simulink model "MPC"  (R2020b)
settings: Solver=ode45  StartTime=0.0  StopTime=1000  RelTol=1e-3  EnableMultiTasking=on
values from neighbouring files (symbols this model uses):
  adingain = [adingain 1 1 1 1 1]    [hwinit.m]
  adinoffs = [adinoffs 0 0 0 0 0]    [hwinit.m]
  daoutgain = 1*[-6]    [hwinit.m]
  daoutoffs = -[-0.0025]    [hwinit.m]
  Theta1_0 = pi    (= 3.14159265359)    [simulation.m]
  Theta2_0 = -pi/2    (= -1.57079632679)    [simulation.m]
  Thetad1_0 = 0    [simulation.m]
  Thetad2_0 = 0    [simulation.m]
undefined symbols (not defined in the file or in its folder): Discrete, h, R, Time
libraries: simulink x4, mpclib x2, ctrlSharedLib x1
settings Model: Creator=rbabuska  LastModifiedBy=fballast
settings DataIOCC: LimitDataPoints=on  SaveFormat=Array  ReturnWorkspaceOutputs=off  SignalLoggingName=sigsOut
settings OptimizationCC: BooleanDataType=off  ExpressionDepthLimit=2147483647  InitFltsAndDblsToZero=on  LifeSpan=inf
settings DebuggingCC: SaveWithParameterizedLinksMsg=none  SignalResolutionControl=TryResolveAllWithWarning  MultiTaskDSMMsg=warning  MultiTaskCondExecSysMsg=none  AllowSymbolicDim=off  StateNameClashWarn=warning  SFUnexpectedBacktrackingDiag=warning  SFNoUnconditionalDefaultTransitionDiag=warning  SFExecutionAtInitializationDiag=none  ArithmeticOperatorsInVariantConditions=warning
settings HardwareCC: ProdBitPerPointer=32  ProdBitPerSizeT=32  ProdBitPerPtrDiffT=32  ProdLargestAtomicFloat=None  ProdIntDivRoundTo=Undefined  ProdEndianess=Unspecified  ProdWordSize=32  ProdHWDeviceType=32-bit Generic  TargetUnknown=on
settings ModelReferenceCC: PropagateSignalLabelsOutOfModel=off
settings SFSimCC: SimUseLocalCustomCode=off  CustomCodeUndefinedFunction=UseInterfaceOnly
settings RTWCC: RTWUseLocalCustomCode=off
settings CodeAppCC: StateflowObjectComments=on
settings GRTTargetCC: TargetFcnLib=ansi_tfl_tmw.mat  TargetLangStandard=C89/C90 (ANSI)  CombineOutputUpdateFcns=off  GRTInterface=on
settings ConfigComp: CovMetricSettings=dw  CovSaveCumulativeToWorkspaceVar=on  CovSaveSingleToWorkspaceVar=on  CovExternalEMLEnable=off

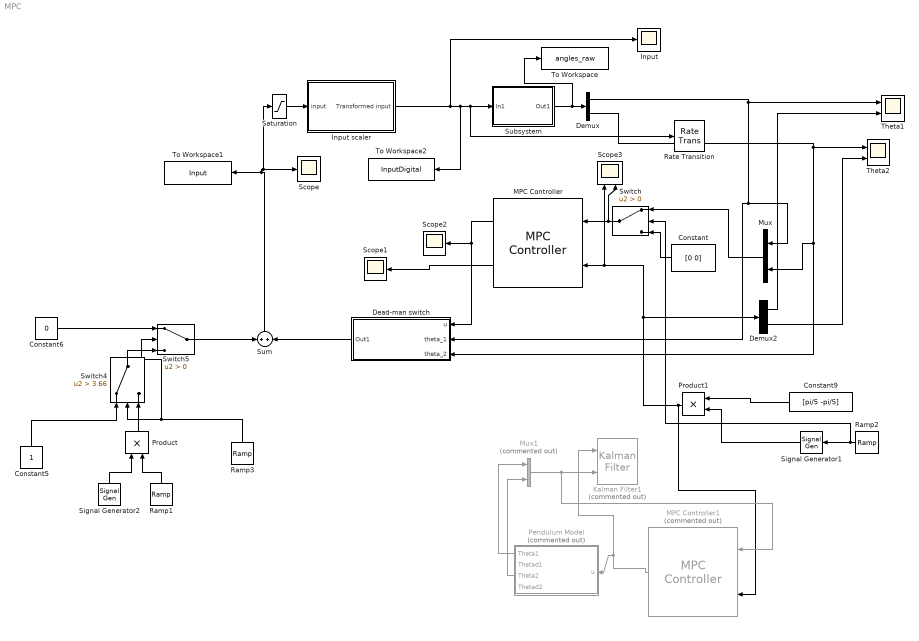
== system MPC ==
  Constant : Constant  Value=[0 0]
  Constant5 : Constant
  Constant6 : Constant  Value=0
  Constant9 : Constant  Value=[pi/5 -pi/5]
  Dead-man switch : Subsystem
  Demux : Demux  Outputs=2
  Demux2 : Demux  Outputs=2
  Input : Scope
  Input scaler : Subsystem
  Kalman Filter1 : ctrlSharedLib/Kalman Filter  Commented=on  TimeDomain=Discrete-Time  UseCurrentEstimator=on  ModelSource=LTI State-Space Variable  ModelSourceVariable=sysd  A=0.95  B=1  C=1  D=0  NumberOfStates=1  NumberOfInputs=1  NumberOfOutputs=1  InitialEstimateSource=Dialog  X0=0  P0=10  UseK=off  UseGH=off  NumberOfProcessNoiseInputs=1  G=eye(4)  TimeInvariantG=on  H=0  TimeInvariantH=on  Q=Q  TimeInvariantQ=on  R=R  TimeInvariantR=on  N=0  TimeInvariantN=on  AddInputPort=on  AddEnablePort=off  OutputEstimatedY=off  OutputP=off  Ts=-1
  MPC Controller : mpclib/MPC Controller  SCDEnableBlockLinearizationSpecification=on  mpcobj=mpc1  is_multiple=0  enable_value=0  return_u0=off  updateMPCinCallerWorkspace=on  md_inport=off  mv_inport=off  uref_inport=off  return_cost=off  return_mvseq=off  return_qpstatus=off  return_xseq=off  return_state=on  return_ovseq=off  state_inport=off  umin_inport=off  umax_inport=off  ymin_inport=off  ymax_inport=off  cc_inport=off  ywt_inport=off  uwt_inport=off  duwt_inport=off  rhoeps_inport=off  pm_inport=off  MaximumP=10  HorizonChoice=FixedHorizon  n_ts=0.01  n_p=40  n_mv=1  n_md=0  n_ud=0  n_mo=2  n_uo=0  BlockDataType=double  SampleTimeInherited=off  switch_inport=off
  MPC Controller1 : mpclib/MPC Controller  Commented=on  SCDEnableBlockLinearizationSpecification=on  mpcobj=mpc1  is_multiple=0  enable_value=0  return_u0=off  updateMPCinCallerWorkspace=on  md_inport=off  mv_inport=off  uref_inport=off  return_cost=off  return_mvseq=off  return_qpstatus=off  return_xseq=off  return_state=off  return_ovseq=off  state_inport=off  umin_inport=off  umax_inport=off  ymin_inport=off  ymax_inport=off  cc_inport=off  ywt_inport=off  uwt_inport=off  duwt_inport=off  rhoeps_inport=off  pm_inport=off  MaximumP=10  HorizonChoice=FixedHorizon  n_ts=0.01  n_p=40  n_mv=1  n_md=0  n_ud=0  n_mo=2  n_uo=0  BlockDataType=double  SampleTimeInherited=off  switch_inport=off
  Mux : Mux  Inputs=2
  Mux1 : Mux  Commented=on  Inputs=2
  Pendulum Model : Subsystem  Commented=on
  Product : Product
  Product1 : Product
  Ramp1 : simulink/Sources/Ramp  slope=0.76  start=0.86  InitialOutput=0
  Ramp2 : simulink/Sources/Ramp  slope=1  start=3  InitialOutput=0
  Ramp3 : simulink/Sources/Ramp  slope=1  start=0  InitialOutput=0
  Rate Transition : RateTransition  OutPortSampleTime=h
  Saturation : Saturate  UpperLimit=1  LowerLimit=-1
  Scope : Scope
  Scope1 : Scope
  Scope2 : Scope
  Scope3 : Scope  NumInputPorts=2
  Signal Generator1 : SignalGenerator  TimeSource=Use external signal  Frequency=0.1
  Signal Generator2 : SignalGenerator  Frequency=1.15
  Subsystem : Subsystem
      mask Display: disp('Rotational\nPendulum')
  Sum : Sum  Inputs=+|+
  Switch : Switch  Criteria=u2 > Threshold
  Switch4 : Switch  Criteria=u2 > Threshold  Threshold=3.66
  Switch5 : Switch  Criteria=u2 > Threshold
  Theta1 : Scope  NumInputPorts=2
  Theta2 : Scope  NumInputPorts=2
  To Workspace : ToWorkspace  VariableName=angles_raw  SaveFormat=Timeseries  SampleTime=-1
  To Workspace1 : ToWorkspace  VariableName=Input  SaveFormat=Timeseries  SampleTime=-1
  To Workspace2 : ToWorkspace  VariableName=InputDigital  SaveFormat=Timeseries  SampleTime=-1
  wires:
  Input scaler/1(Transformed input) -> To Workspace2/1, Rate Transition/1, Subsystem/1(In1), Input/1
  Subsystem/1(Out1) -> To Workspace/1, Demux/1
  Demux/1 -> Theta1/1, Dead-man switch/2(theta_1), Mux/1
  Demux/2 -> Dead-man switch/3(theta_2), Mux/2, Theta2/1
  MPC Controller/1 -> Scope2/1, Dead-man switch/1(u)
  Signal Generator1/1 -> Product1/2
  Demux2/1 -> Theta1/2
  Demux2/2 -> Theta2/2
  Ramp2/1 -> Switch/2, Signal Generator1/1
  Constant9/1 -> Product1/1
  Sum/1 -> To Workspace1/1, Saturation/1, Scope/1
  Dead-man switch/1(Out1) -> Sum/2
  Signal Generator2/1 -> Product/1
  Ramp1/1 -> Product/2
  Product/1 -> Switch4/3
  Constant5/1 -> Switch4/1
  Ramp3/1 -> Switch5/2, Switch4/2
  Switch5/1 -> Sum/1
  Constant6/1 -> Switch5/1
  Switch4/1 -> Switch5/3
  Pendulum Model/1(Theta1) -> Mux1/1
  Pendulum Model/3(Theta2) -> Mux1/2
  MPC Controller1/1 -> Kalman Filter1/1, Pendulum Model/1(u)
  Switch/1 -> MPC Controller/1, Scope3/2
  Constant/1 -> Switch/3
  MPC Controller/2 -> Scope1/1
  Product1/1 -> MPC Controller1/2, MPC Controller/2, Scope3/1, Demux2/1
  Mux/1 -> Switch/1
  Saturation/1 -> Input scaler/1(input)
  Mux1/1 -> MPC Controller1/1, Kalman Filter1/2

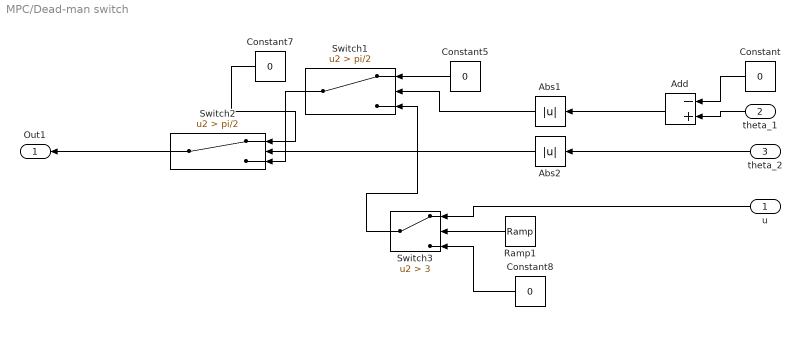
== system MPC/Dead-man switch ==
  u : Inport
  theta_1 : Inport  Port=2
  theta_2 : Inport  Port=3
  Abs1 : Abs
  Abs2 : Abs
  Add : Sum  Inputs=-+
  Constant{,5,7..8} (4 alike) : Constant  Value=0
  Ramp1 : simulink/Sources/Ramp  slope=1  start=0  InitialOutput=0
  Switch1 : Switch  Criteria=u2 > Threshold  Threshold=pi/2
  Switch2 : Switch  Criteria=u2 > Threshold  Threshold=pi/2
  Switch3 : Switch  Criteria=u2 > Threshold  Threshold=3
  Out1 : Outport
  wires:
  Switch3/1 -> Switch1/3
  Ramp1/1 -> Switch3/2
  Abs2/1 -> Switch2/2
  Abs1/1 -> Switch1/2
  Constant5/1 -> Switch1/1
  Constant7/1 -> Switch2/1
  Switch1/1 -> Switch2/3
  Constant8/1 -> Switch3/3
  theta_2/1 -> Abs2/1
  u/1 -> Switch3/1
  Switch2/1 -> Out1/1
  theta_1/1 -> Add/2
  Add/1 -> Abs1/1
  Constant/1 -> Add/1

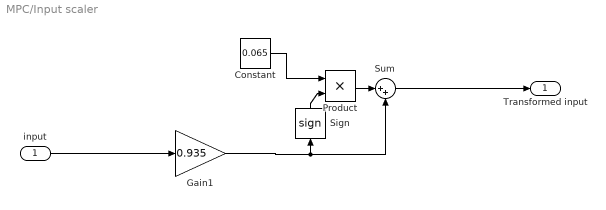
== system MPC/Input scaler ==
  input : Inport
  Constant : Constant  Value=0.065
  Gain1 : Gain  Gain=0.935
  Product : Product
  Sign : Signum
  Sum : Sum  Inputs=|++
  Transformed input : Outport
  wires:
  Gain1/1 -> Sum/2, Sign/1
  Constant/1 -> Product/1
  Sign/1 -> Product/2
  Sum/1 -> Transformed input/1
  Product/1 -> Sum/1
  input/1 -> Gain1/1

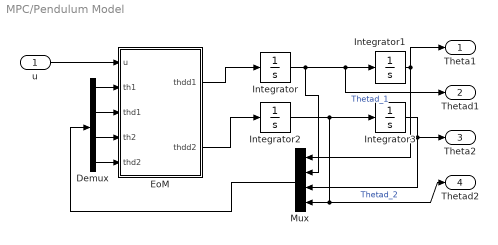
== system MPC/Pendulum Model ==
  u : Inport
  Demux : Demux
  EoM : MATLAB Function  TreatAsAtomicUnit=on
  Integrator : Integrator  InitialCondition=Thetad1_0  ContinuousStateAttributes='Theta1'
  Integrator1 : Integrator  InitialCondition=Theta1_0  ContinuousStateAttributes='Theta1'
  Integrator2 : Integrator  InitialCondition=Thetad2_0  ContinuousStateAttributes='Theta1'
  Integrator3 : Integrator  InitialCondition=Theta2_0  ContinuousStateAttributes='Theta1'
  Mux : Mux
  Theta1 : Outport
  Thetad1 : Outport  Port=2
  Theta2 : Outport  Port=3
  Thetad2 : Outport  Port=4
  wires:
  Integrator1/1 -> Mux/1, Theta1/1
  Integrator/1 -> Mux/2, Integrator1/1, Thetad1/1  "Thetad_1"
  EoM/2(thdd2) -> Integrator2/1
  Integrator2/1 -> Thetad2/1, Mux/4, Integrator3/1  "Thetad_2"
  Integrator3/1 -> Theta2/1, Mux/3
  u/1 -> EoM/1(u)
  EoM/1(thdd1) -> Integrator/1
  Demux/1 -> EoM/2(th1)
  Demux/2 -> EoM/3(thd1)
  Demux/3 -> EoM/4(th2)
  Demux/4 -> EoM/5(thd2)
  Mux/1 -> Demux/1

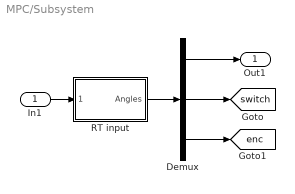
== system MPC/Subsystem ==
  In1 : Inport
  Demux : Demux  Outputs=[2 4 1]
  RT input : Subsystem  mask{Ts=h, channels=[6 7]}
      mask prompts: Ts "Sample time [s]:"; channels "Channels to read (e.g., [6 7])"
      mask init:
      | hwinit;
      | 
      | % initialize FPGA
      | fugihandle = fugiboard('Open', 'Pendulum1');
      | fugihandle.WatchdogTimeout = 0.5;
      | fugiboard('SetParams', fugihandle);
      | fugiboard('Write', fugihandle, 0, 0, 0, 0);  % dummy write to sync interface board
      | fugiboard('Write', fugihandle, 5, 1, 0, 0);  % reset position, activate relay
      | data = fugiboard('Read', fugihandle);        % get version info from FPGA
      | % model = bitshift(data(1), -5); 
      | % version = bitand(data(1), 31);
      | % disp(sprintf('FPGA setup %d, version %d', model, version)); % for the B&P it should say 1 1, or else there is a problem
      | fugiboard('Write', fugihandle, 0, 1, 0, 0);  % end reset
      | pause(0.1);                         % give relay some time to respond
      mask Display: disp('Rotational\nPendulum')
  Out1 : Outport
  tag scope: enc=global, switch=global
  wires:
  RT input/1(Angles) -> Demux/1
  Demux/1 -> Out1/1
  Demux/2 -> [switch]
  Demux/3 -> [enc]
  In1/1 -> RT input/1(Motors)

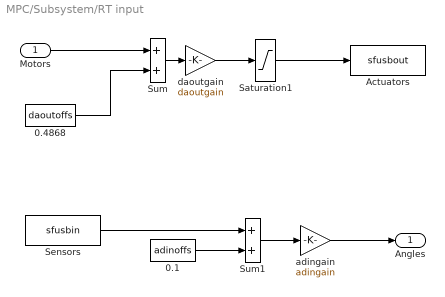
== system MPC/Subsystem/RT input ==
  Motors : Inport
  0.1 : Constant  Value=adinoffs
  0.4868 : Constant  Value=daoutoffs
  Actuators : S-Function  FunctionName=sfusbout  Parameters=Ts, fugihandle  SFunctionDeploymentMode=off  EnableBusSupport=off
  Saturation1 : Saturate  UpperLimit=10  LowerLimit=-10
  Sensors : S-Function  FunctionName=sfusbin  Parameters=Ts, fugihandle, channels  SFunctionDeploymentMode=off  EnableBusSupport=off
  Sum : Sum  InputSameDT=on  SaturateOnIntegerOverflow=on  OutDataTypeStr=Inherit: Same as first input
  Sum1 : Sum  InputSameDT=on  SaturateOnIntegerOverflow=on  OutDataTypeStr=Inherit: Same as first input
  adingain : Gain  Gain=adingain  SaturateOnIntegerOverflow=on  OutDataTypeStr=Inherit: Same as input  ParamDataTypeStr=Inherit: Same as input
  daoutgain : Gain  Gain=daoutgain  SaturateOnIntegerOverflow=on  OutDataTypeStr=Inherit: Same as input  ParamDataTypeStr=Inherit: Same as input
  Angles : Outport
  wires:
  Sum/1 -> daoutgain/1
  0.4868/1 -> Sum/2
  Motors/1 -> Sum/1
  Sum1/1 -> adingain/1
  0.1/1 -> Sum1/2
  adingain/1 -> Angles/1
  Saturation1/1 -> Actuators/1
  daoutgain/1 -> Saturation1/1
  Sensors/1 -> Sum1/1

== matlab function MPC/Pendulum Model/EoM ==
  data: u input; thdd1 output; th1 input; thd1 input; th2 input; thd2 input; model_par parameter; thdd2 output
function [thdd1, thdd2] = fcn(u, th1, thd1, th2, thd2, model_par)
thdd1 = -model_par.a11*thd1 - model_par.a12 * u;
F = -model_par.c2*model_par.l1*model_par.m2*sin(thd2)*thd1^2 - model_par.b2*thd2 + model_par.c2*model_par.g*model_par.m2*sin(th1 + th2);
M21 = model_par.m2*model_par.c2^2 + model_par.l1*model_par.m2*cos(thd2)*model_par.c2 + model_par.J2;
M22 = model_par.m2*model_par.c2^2 + model_par.J2;
thdd2 = F/M22 - M21/M22 * thdd1;
